simulink model "Autopilot_wk1"  (R2026a)
settings: Solver=ode4  FixedStep=0.001
settings Model: Creator=anirudhbohare  LastModifiedBy=s1808

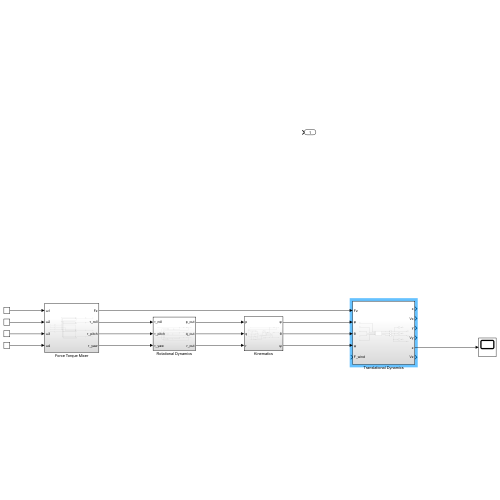
[thumbnail: Simulink's stored preview of the top-level diagram]
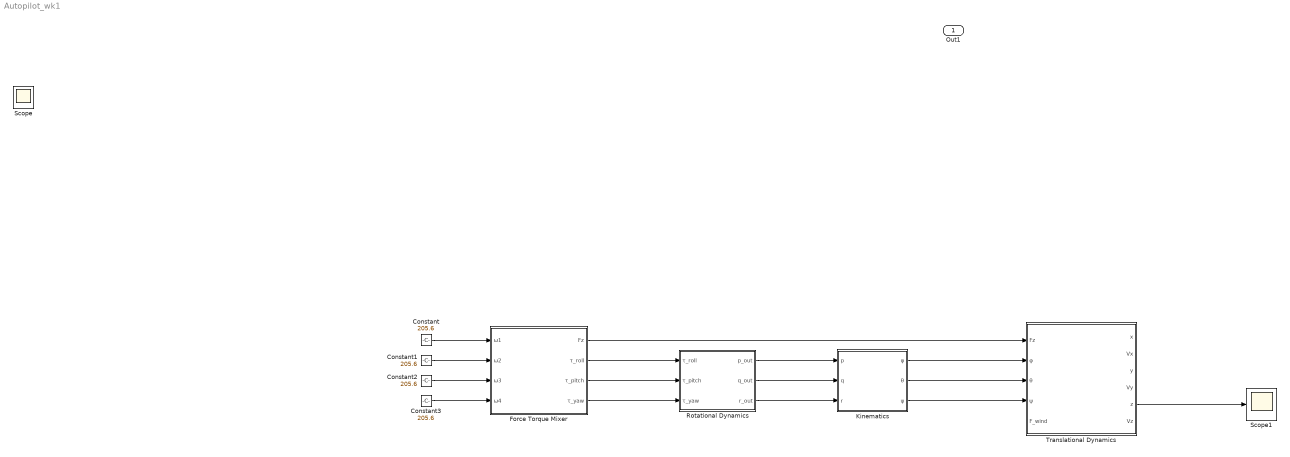
== system Autopilot_wk1 ==
  Constant{,1..3} (4 alike) : Constant  Value=205.6
  Force Torque Mixer : Subsystem
  Kinematics : Subsystem
  Rotational Dynamics : Subsystem
  Scope1 : Scope
      settings: ActiveDisplayYMinimum=0.15200151199465087  ActiveDisplayYMaximum=0.15236860241057831
  Translational Dynamics : Subsystem
  Out1 : Outport
  Scope : Scope
      settings: ActiveDisplayYMinimum=-1  ActiveDisplayYMaximum=1
  wires:
  Rotational Dynamics/1(p_out) -> Kinematics/1(p)
  Rotational Dynamics/2(q_out) -> Kinematics/2(q)
  Rotational Dynamics/3(r_out) -> Kinematics/3(r)
  Kinematics/1(φ) -> Translational Dynamics/2(φ)
  Kinematics/2(θ) -> Translational Dynamics/3(θ)
  Kinematics/3(ψ) -> Translational Dynamics/4(ψ)
  Force Torque Mixer/1(Fz) -> Translational Dynamics/1(Fz)
  Force Torque Mixer/3(τ_pitch) -> Rotational Dynamics/2(τ_pitch)
  Force Torque Mixer/4(τ_yaw) -> Rotational Dynamics/3(τ_yaw)
  Force Torque Mixer/2(τ_roll) -> Rotational Dynamics/1(τ_roll)
  Translational Dynamics/5(z) -> Scope1/1
  Constant3/1 -> Force Torque Mixer/4(ω4)
  Constant2/1 -> Force Torque Mixer/3(ω3)
  Constant1/1 -> Force Torque Mixer/2(ω2)
  Constant/1 -> Force Torque Mixer/1(ω1)

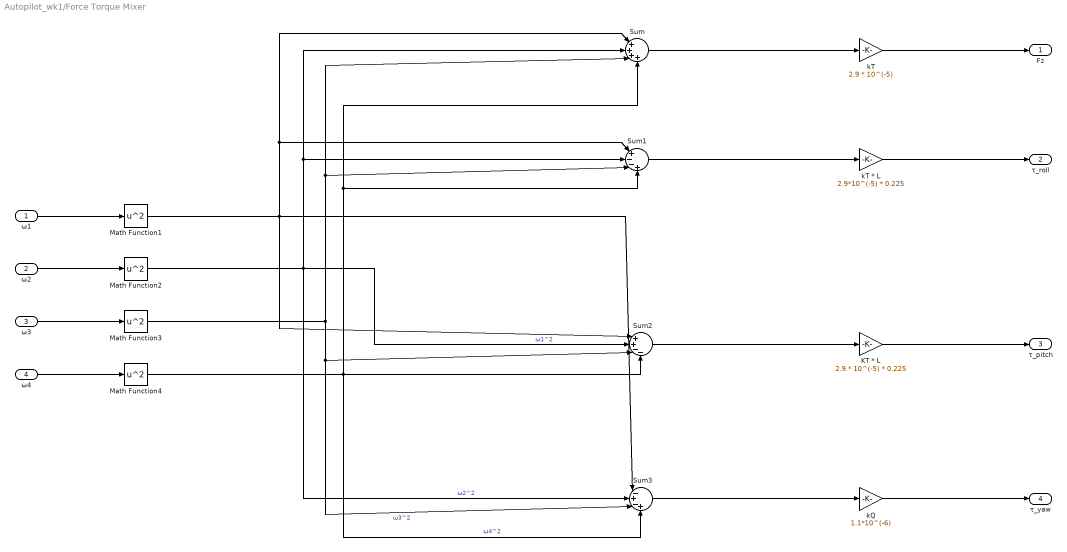
== system Autopilot_wk1/Force Torque Mixer ==
  ω1 : Inport
  ω2 : Inport  Port=2
  ω3 : Inport  Port=3
  ω4 : Inport  Port=4
  KT * L : Gain  Gain=2.9 * 10^(-5) * 0.225
  Math Function{1..4} (4 alike) : Math  Operator=square
  Sum : Sum  Inputs=|++++
  Sum1 : Sum  Inputs=|+--+
  Sum2 : Sum  Inputs=|++--
  Sum3 : Sum  Inputs=|-+-+
  kQ : Gain  Gain=1.1*10^(-6)
  kT : Gain  Gain=2.9 * 10^(-5)
  kT * L : Gain  Gain=2.9*10^(-5) * 0.225
  Fz : Outport
  τ_roll : Outport  Port=2
  τ_pitch : Outport  Port=3
  τ_yaw : Outport  Port=4
  wires:
  ω1/1 -> Math Function1/1
  ω2/1 -> Math Function2/1
  ω3/1 -> Math Function3/1
  ω4/1 -> Math Function4/1
  Math Function2/1 -> Sum2/2, Sum3/2, Sum/2, Sum1/2  "ω2^2"
  Math Function3/1 -> Sum3/3, Sum2/3, Sum/3, Sum1/3  "ω3^2"
  Math Function4/1 -> Sum3/4, Sum2/4, Sum1/4, Sum/4  "ω4^2"
  Math Function1/1 -> Sum3/1, Sum2/1, Sum1/1, Sum/1  "ω1^2"
  Sum/1 -> kT/1
  Sum1/1 -> kT * L/1
  Sum2/1 -> KT * L/1
  Sum3/1 -> kQ/1
  kQ/1 -> τ_yaw/1
  KT * L/1 -> τ_pitch/1
  kT * L/1 -> τ_roll/1
  kT/1 -> Fz/1

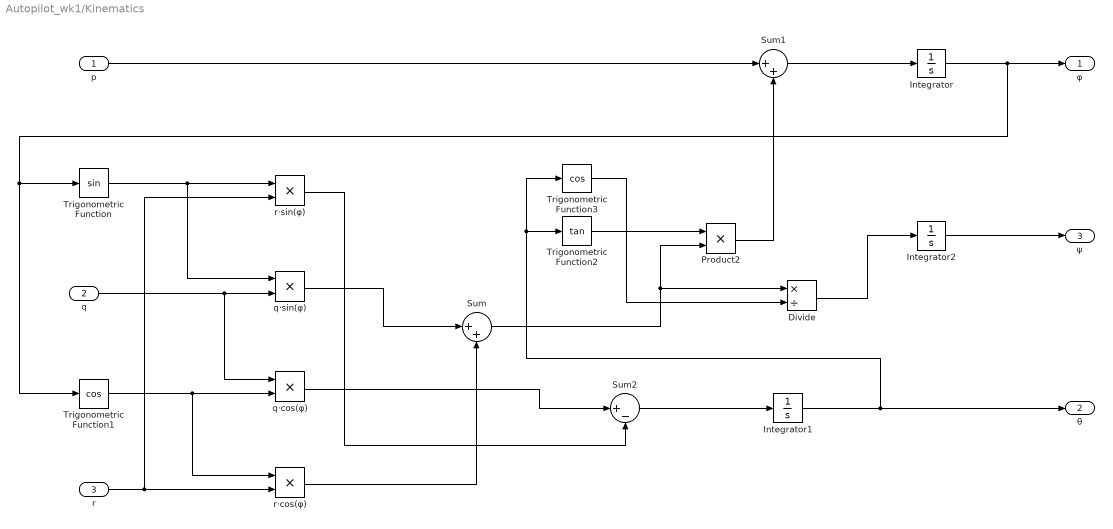
== system Autopilot_wk1/Kinematics ==
  p : Inport
  q : Inport  Port=2
  r : Inport  Port=3
  Divide : Product  Inputs=*/
  Integrator : Integrator
  Integrator1 : Integrator
  Integrator2 : Integrator
  Product2 : Product
  Sum : Sum  Inputs=|++
  Sum1 : Sum  Inputs=|++
  Sum2 : Sum  Inputs=|+-
  Trigonometric Function : Trigonometry
  Trigonometric Function1 : Trigonometry  Operator=cos
  Trigonometric Function2 : Trigonometry  Operator=tan
  Trigonometric Function3 : Trigonometry  Operator=cos
  q·cos(φ) : Product
  q·sin(φ) : Product
  r·cos(φ) : Product
  r·sin(φ) : Product
  φ : Outport
  θ : Outport  Port=2
  ψ : Outport  Port=3
  wires:
  Trigonometric Function/1 -> q·sin(φ)/1, r·sin(φ)/1
  q/1 -> q·cos(φ)/1, q·sin(φ)/2
  Trigonometric Function1/1 -> r·cos(φ)/1, q·cos(φ)/2
  r/1 -> r·sin(φ)/2, r·cos(φ)/2
  q·sin(φ)/1 -> Sum/1
  r·cos(φ)/1 -> Sum/2
  Sum/1 -> Divide/1, Product2/2
  Trigonometric Function2/1 -> Product2/1
  Product2/1 -> Sum1/2
  p/1 -> Sum1/1
  Sum1/1 -> Integrator/1
  Integrator/1 -> Trigonometric Function1/1, Trigonometric Function/1, φ/1
  q·cos(φ)/1 -> Sum2/1
  r·sin(φ)/1 -> Sum2/2
  Sum2/1 -> Integrator1/1
  Integrator1/1 -> Trigonometric Function2/1, Trigonometric Function3/1, θ/1
  Trigonometric Function3/1 -> Divide/2
  Divide/1 -> Integrator2/1
  Integrator2/1 -> ψ/1

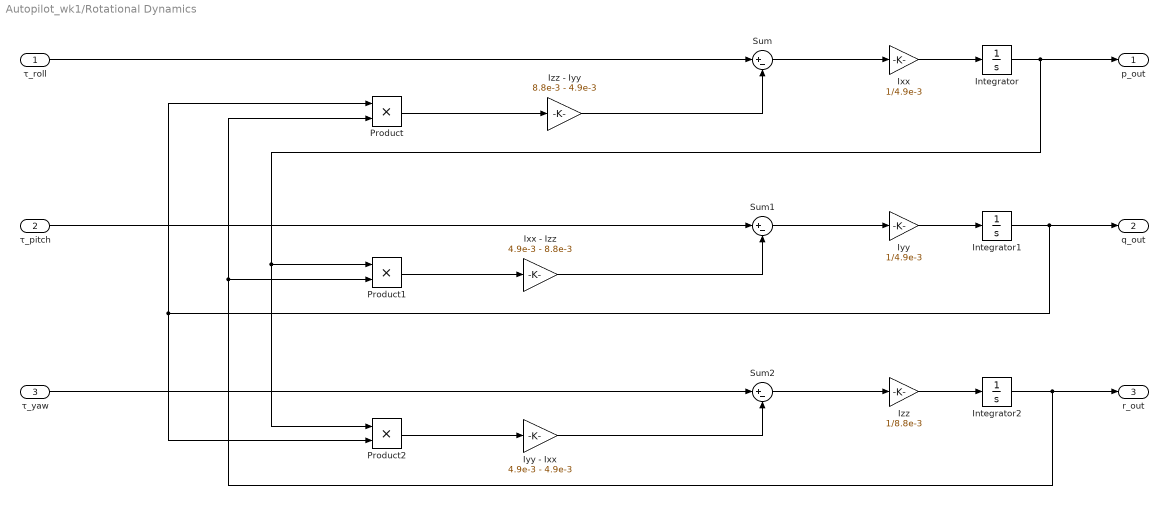
== system Autopilot_wk1/Rotational Dynamics ==
  τ_roll : Inport
  τ_pitch : Inport  Port=2
  τ_yaw : Inport  Port=3
  Integrator : Integrator
  Integrator1 : Integrator
  Integrator2 : Integrator
  Ixx : Gain  Gain=1/4.9e-3
  Ixx - Izz : Gain  Gain=4.9e-3 - 8.8e-3
  Iyy : Gain  Gain=1/4.9e-3
  "Iyy - Ixx " : Gain  Gain=4.9e-3 - 4.9e-3
  Izz : Gain  Gain=1/8.8e-3
  Izz - Iyy : Gain  Gain=8.8e-3 - 4.9e-3
  Product : Product
  Product1 : Product
  Product2 : Product
  Sum : Sum  Inputs=|+-
  Sum1 : Sum  Inputs=|+-
  Sum2 : Sum  Inputs=|+-
  p_out : Outport
  q_out : Outport  Port=2
  r_out : Outport  Port=3
  wires:
  τ_roll/1 -> Sum/1
  Integrator1/1 -> q_out/1, Product2/2, Product/1
  Integrator2/1 -> r_out/1, Product1/2, Product/2
  Product/1 -> Izz - Iyy/1
  Izz - Iyy/1 -> Sum/2
  Sum/1 -> Ixx/1
  Ixx/1 -> Integrator/1
  Integrator/1 -> p_out/1, Product2/1, Product1/1
  Product1/1 -> Ixx - Izz/1
  Ixx - Izz/1 -> Sum1/2
  τ_pitch/1 -> Sum1/1
  Sum1/1 -> Iyy/1
  Iyy/1 -> Integrator1/1
  Product2/1 -> "Iyy - Ixx "/1
  "Iyy - Ixx "/1 -> Sum2/2
  τ_yaw/1 -> Sum2/1
  Sum2/1 -> Izz/1
  Izz/1 -> Integrator2/1

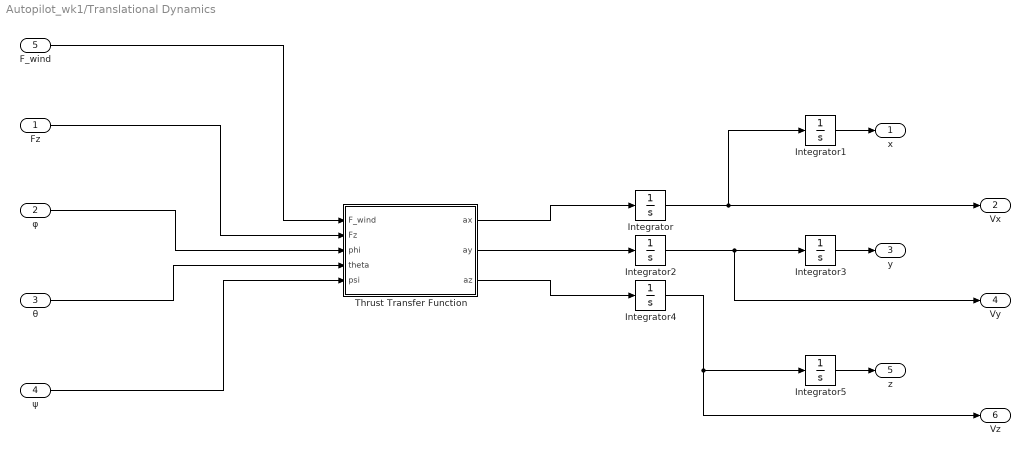
== system Autopilot_wk1/Translational Dynamics ==
  Fz : Inport
  φ : Inport  Port=2
  θ : Inport  Port=3
  ψ : Inport  Port=4
  F_wind : Inport  Port=5  PortDimensions=[3 1]
  Integrator{,1..5} (6 alike) : Integrator
  Thrust Transfer Function : MATLAB Function  TreatAsAtomicUnit=on
  x : Outport
  Vx : Outport  Port=2
  y : Outport  Port=3
  Vy : Outport  Port=4
  z : Outport  Port=5
  Vz : Outport  Port=6
  wires:
  Fz/1 -> Thrust Transfer Function/2(Fz)
  φ/1 -> Thrust Transfer Function/3(phi)
  θ/1 -> Thrust Transfer Function/4(theta)
  ψ/1 -> Thrust Transfer Function/5(psi)
  Thrust Transfer Function/2(ay) -> Integrator2/1
  Thrust Transfer Function/1(ax) -> Integrator/1
  Thrust Transfer Function/3(az) -> Integrator4/1
  Integrator/1 -> Integrator1/1, Vx/1
  Integrator2/1 -> Vy/1, Integrator3/1
  Integrator4/1 -> Vz/1, Integrator5/1
  Integrator1/1 -> x/1
  Integrator3/1 -> y/1
  Integrator5/1 -> z/1
  F_wind/1 -> Thrust Transfer Function/1(F_wind)

== matlab function Autopilot_wk1/Translational Dynamics/Thrust Transfer Function ==
  data: F_wind input; Fz input; ax output; phi input; theta input; psi input; ay output; az output
function [ax, ay, az] = fcn(F_wind, Fz, phi, theta, psi)

m = 0.5;   % kg
g = 9.81;  % m/s²

% Rotation matrix R (body → world)
R = [cos(theta)*cos(psi), ...
    sin(phi)*sin(theta)*cos(psi) - cos(phi)*sin(psi), ...
    cos(phi)*sin(theta)*cos(psi) + sin(phi)*sin(psi);

    cos(theta)*sin(psi), ...
    sin(phi)*sin(theta)*sin(psi) + cos(phi)*cos(psi), ...
    cos(phi)*sin(theta)*sin(psi) - sin(phi)*cos(psi);

    -sin(theta), ...
    sin(phi)*cos(theta), ...
    cos(phi)*cos(theta)];

% Thrust in body frame (opposes +z/down direction)
F_body = [0;0;-Fz];

% Rotate to world frame, add gravity
F_world = R*F_body + F_wind + [0;0;m*g];

% Accelerations
ax=F_world(1)/m;
ay=F_world(2)/m;
az=F_world(3)/m;
end
